simulink model "RocketAirBrake_Simulation_Alan"  (R2018b)
settings: Solver=FixedStepAuto  StartTime=0.0  StopTime=30  FixedStep=0.001  RelTol=1e-3
libraries: embdlinuxlib x6
(part 3 of 3)

== matlab function RocketAirBrake_Simulation_Alan/Rocket Dynamics/MATLAB Function1 ==
  data: airbrake_angle input; Cd output
function Cd = dragTF(airbrake_angle)

%%%%%%%%%%%%%% REPLACE THIS WITH BETTER MODEL BASED ON CFD %%%%%%%%%%%%%%%%
% Also add mach number dependency

Cd_rocket = 0.4; % Coefficient of drag of rocket
A_ref = 0.010751315458748; % [m^2] rocket reference area
Cd_flat_plate = 1.28; % https://www.grc.nasa.gov/www/k-12/airplane/shaped.html
TF = 3.888e-3; % Linear fit of area to angle from Solidworks data

A_flat_plate = TF*airbrake_angle; % Calculate exposed area
Cd = Cd_rocket + Cd_flat_plate*A_flat_plate/A_ref; % Calculate Drag Coefficient

== matlab function RocketAirBrake_Simulation_Alan/MATLAB Function1 ==
  data: error input; Angle_out output; step_in input; step_out output; Angle_in input
function [Angle_out, step_out]= fcn(error, step_in,Angle_in)
%#codegen,
GR = 2.5;
if (error > 0)
    correction = -1.8; 
elseif (error < 0)
    correction = 1.8;
else
    correction = 0;
end
if((Angle_in == 90) && (correction > 0))
    Angle_out = Angle_in;
    step_out = step_in; 
    return;
elseif((Angle_in == 0) && (correction < 0))
    Angle_out = Angle_in;
    step_out = step_in;
    return;
else
step_out = step_in + correction;
shaft_angle = step_out*1.8; 
Angle_out = shaft_angle*GR; 
Angle_out = min(max(0,Angle_out),90);
end
% Motor_Angle = AirBrake_Angle*GR;
% %if error is postive, rocket is undershooting, decrease area
% %if error is negative, rocket is overshooting, increase area
% Steps = Motor_Angle/1.8;
